simulink model "Utkarsh_2005574_R_W3_P3"  (R2021a)
settings: Solver=VariableStepAuto  StartTime=0.0  StopTime=10.0  RelTol=1e-3
undefined symbols (not defined in the file): g, m, mu, Rr, slip, v0
settings Model: Creator=Utkarsh Anand  LastModifiedBy=Utkarsh Anand

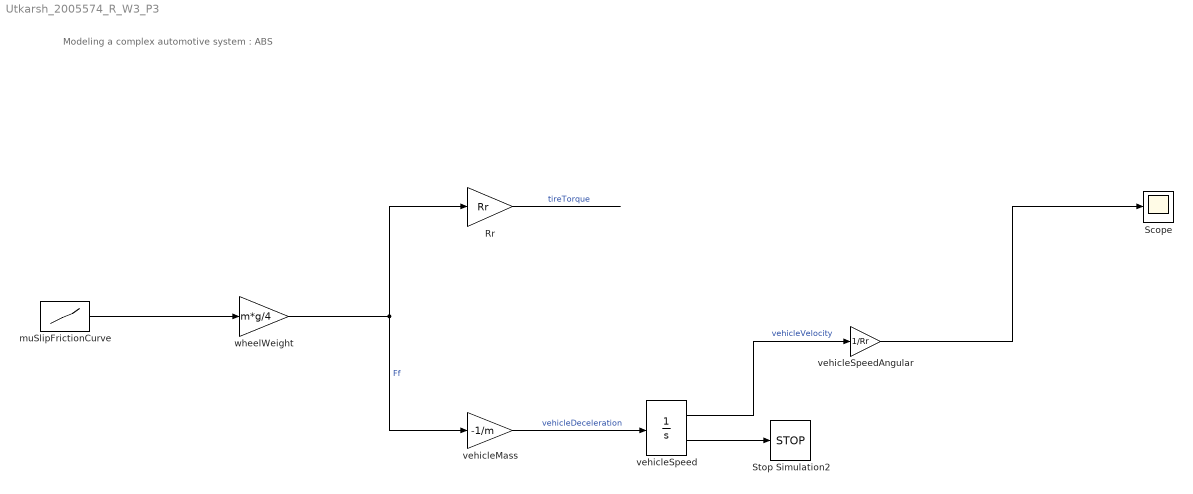
== system Utkarsh_2005574_R_W3_P3 ==
  note: Modeling a complex automotive system : ABS
  Rr : Gain  Gain=Rr
  Scope : Scope
  Stop Simulation2 : Stop
  muSlipFrictionCurve : Lookup_n-D  NumberOfTableDimensions=1  BreakpointsForDimension1=slip  Table=mu  SaturateOnIntegerOverflow=on  InputSameDT=on
  vehicleMass : Gain  Gain=-1/m
  vehicleSpeed : Integrator  InitialCondition=v0  LimitOutput=on  UpperSaturationLimit=1000  LowerSaturationLimit=0  ShowSaturationPort=on
  vehicleSpeedAngular : Gain  Gain=1/Rr
  wheelWeight : Gain  Gain=m*g/4
  wires:
  muSlipFrictionCurve/1 -> wheelWeight/1
  wheelWeight/1 -> Rr/1, vehicleMass/1  "Ff"
  Rr/1 -> ?  "tireTorque"
  vehicleMass/1 -> vehicleSpeed/1  "vehicleDeceleration"
  vehicleSpeed/1 -> vehicleSpeedAngular/1  "vehicleVelocity"
  vehicleSpeedAngular/1 -> Scope/1
  vehicleSpeed/2 -> Stop Simulation2/1
